simulink model "TwoLevelConverterIdealExample_Pejovic"  (R2023b)
settings: Solver=FixedStepDiscrete  StartTime=0.0  StopTime=100/fsw  MaxStep=1e-4  RelTol=1e-6  AbsTol=1e-6
PreLoadFcn:
  | ts = 1e-5; % local solver sample period
  | fsw = 1e3; % switching frequency
undefined symbols (not defined in the file): DiscIntNeverNeededParam, subcycleFactor
libraries: nesl_utility x53, fl_lib x52, ee_lib x16, simulink x12, fpga_utils_lib x12, eePwmGeneratorTwoLevel x1
(part 1 of 2)
CloseFcn:
  | clear ts fsw;
settings Model: DataTypeOverride=Off  Creator=The MathWorks, Inc.  LastModifiedBy=promero
settings SolverCC: AutoScaleAbsTol=off  AlgebraicLoopSolver=TrustRegion
settings DataIOCC: LimitDataPoints=on  SaveFormat=StructureWithTime  SaveOutput=off  DSMLogging=off  SaveTime=off  ReturnWorkspaceOutputs=off
settings OptimizationCC: BlockReduction=off  ConditionallyExecuteInputs=off  DefaultParameterBehavior=Inlined  OptimizeBlockIOStorage=off  BufferReuse=off  GlobalBufferReuse=off  ExpressionFolding=off  LocalBlockOutputs=off  OptimizeDataStoreBuffers=off  BusAssignmentInplaceUpdate=off
settings DebuggingCC: AlgebraicLoopMsg=error  SolverPrmCheckMsg=warning  SingleTaskRateTransMsg=error  UnconnectedInputMsg=warning  UnconnectedOutputMsg=warning  UnconnectedLineMsg=warning  AllowSymbolicDim=off  PregeneratedLibrarySubsystemCodeDiagnostic=none  SFUnexpectedBacktrackingDiag=warning  SFNoUnconditionalDefaultTransitionDiag=warning  SFExecutionAtInitializationDiag=none  ArithmeticOperatorsInVariantConditions=warning
settings HardwareCC: ProdBitPerPointer=32  ProdBitPerSizeT=32  ProdBitPerPtrDiffT=32  ProdLargestAtomicFloat=None  ProdIntDivRoundTo=Undefined  ProdEndianess=Unspecified  ProdWordSize=32  ProdHWDeviceType=ASIC/FPGA->ASIC/FPGA  TargetBitPerPointer=64  TargetBitPerSizeT=64  TargetBitPerPtrDiffT=64  TargetLongLongMode=on  TargetIntDivRoundTo=Zero  TargetEndianess=LittleEndian  TargetWordSize=64  TargetHWDeviceType=Custom Processor->MATLAB Host Computer  ProdEqTarget=off
settings ModelReferenceCC: EnableRefExpFcnMdlSchedulingChecks=on  PropagateSignalLabelsOutOfModel=off
settings SFSimCC: SimUseLocalCustomCode=off  CustomCodeUndefinedFunction=UseInterfaceOnly
settings RTWCC: RTWUseLocalCustomCode=off  RTWCompilerOptimization=on
settings CodeAppCC: StateflowObjectComments=on
settings GRTTargetCC: TargetLangStandard=C89/C90 (ANSI)
settings ConfigComp: CovMetricSettings=dw  CovSaveCumulativeToWorkspaceVar=on  CovSaveSingleToWorkspaceVar=on  CovExternalEMLEnable=off  CovSFcnEnable=off
settings SimscapeCC: SimscapeNormalizeSystem=off  SimscapeNominalValues="[{\"value\":\"10\",\"unit\":\"V\"},{\"value\":\"1\",\"unit\":\"A\"},{\"value\":\"10\",\"unit\":\"N*m\"},{\"value\":\"10\",\"unit\":\"bar\"},{\"value\":\"100\",\"unit\":\"kJ/kg\"},{\"value\":\"1\",\"unit\":\"kW\"},{\"value\":\"300\",\"unit\":\"K\"},{\"value\":\"100\",\"unit\":\"cm^3/s\"},{\"value\":\"1\",\"unit\":\"kN\"},{\"value\":\"1\",\"unit\":\"g/cm^3\"},{\"value\":\"1\",\"unit\":\"l\"},{\"value\":\"1\",\"unit\":\"cm^2\"},{\"value\":\"60\",\"unit\":\"Hz\"}]"  SimscapeLogType=all

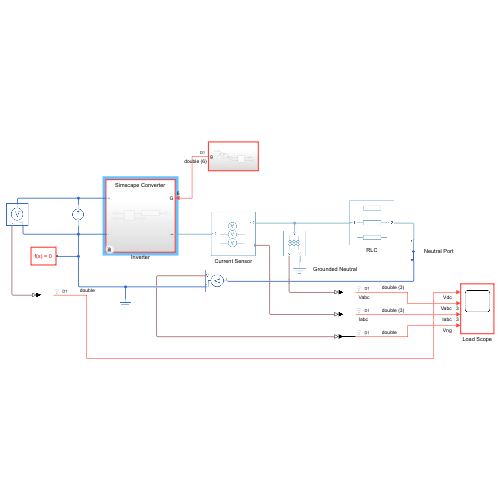
[thumbnail: Simulink's stored preview of the top-level diagram]
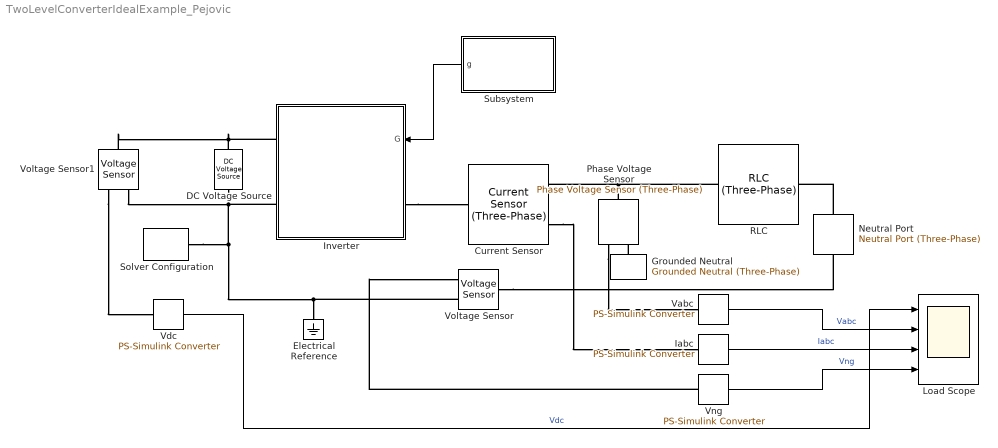
== system TwoLevelConverterIdealExample_Pejovic ==
  Current Sensor : ee_lib/Sensors & Transducers/Current Sensor (Three-Phase)
  DC Voltage Source : fl_lib/Electrical/Electrical Sources/DC Voltage Source  v0=400 V
  Electrical Reference : fl_lib/Electrical/Electrical Elements/Electrical Reference
  Grounded Neutral : ee_lib/Connectors & References/Grounded Neutral (Three-Phase)
  Iabc : nesl_utility/PS-Simulink Converter  PhysicalDomain=network_engine_domain  SubClassName=ps_output  LeftPortType=input  RightPortType=output  PseudoPeriodic=off  Frequencies=[]  VectorFormat=1-D array  Unit=1  AffineConversion=off
  Inverter : Subsystem  Variant=on  VariantControlMode=label  VariantControl=Choice  LabelModeActiveChoice=SimscapeConv
  Load Scope : Scope  NumInputPorts=4
  Neutral Port : ee_lib/Connectors & References/Neutral Port (Three-Phase)  G_parasitic=1e-12 1/Ohm
      settings: InternalSimscapePortConfiguration="{\"Bottom\":[],\"Left\":[{\"id\":\"N\",\"label\":\"~\",\"type\":\"foundation.electrical.three_phase\"}],\"Right\":[{\"id\":\"n\",\"label\":\"n\",\"type\":\"foundation.electrical.electrical\"}],\"Top\":[]}"
  Phase Voltage Sensor : ee_lib/Sensors & Transducers/Phase Voltage Sensor (Three-Phase)
  RLC : ee_lib/Passive/RLC Assemblies/RLC (Three-Phase)  component_structure=4  R=0.1 Ohm  L=0.001 H  C=1e-6 F  R_parasitic=1e-6 Ohm  G_parasitic=1e-6 1/Ohm  IL_specify=on  IL_priority=High  IL=[ 0 0 0 ] A  IL_nominal_specify=off  IL_nominal_unit=A  IL_nominal_value=1  VC_specify=on  VC_priority=High  VC=[ 0 0 0 ] V  VC_nominal_specify=off  VC_nominal_unit=V  VC_nominal_value=1
      settings: InternalSimscapePortConfiguration="{\"Bottom\":[],\"Left\":[{\"id\":\"N1\",\"label\":\"~1\",\"type\":\"foundation.electrical.three_phase\"}],\"Right\":[{\"id\":\"N2\",\"label\":\"~2\",\"type\":\"foundation.electrical.three_phase\"}],\"Top\":[]}"
  Solver Configuration : nesl_utility/Solver Configuration  PhysicalDomain=network_engine_domain  SubClassName=solver  LeftPortType=input  RightPortType=generic  Tones=[]  Harmonics=[]  SimulateNoise=off  Profile=off  UseLocalSampling=off  EnableSwitchedLinearOptims=on  FrequencyDomain=off  UseCCode=off  RelTol=0.001  AbsTol=1e-06  MinStep=1e-09  ToWorkspace=off  RevertToSquareIcSolve=off  NumHomotopyIterations=100  PhasorMode=off  PhasorModeNumHarmonics=1  ConsistencySolver=NEWTON_FTOL  IndexReductionMethod=DerivativeReplacement  DoDC=off  ResidualTolerance=1e-09  ConsistencyTolSource=GLOBAL  ConsistencyAbsTol=0.001  ConsistencyRelTol=0.001  ConsistencyTolFactor=0.001  UseLocalSolver=on  LocalSolverChoice=NE_BACKWARD_EULER_ADVANCER  ResolveIndetEquations=on  FunctionEvalNumThread=1  LocalSolverSampleTime=ts  DoFixedCost=off  MaxNonlinIter=3  MaxModeIter=2  ComputeImpulses=off  ImpulseIterations=2  LinearAlgebra=Sparse  LinearAlgebraNumThread=0  EquationFormulation=NE_TIME_EF  DelaysMemoryBudget=1024  AutomaticFiltering=on  FilteringTimeConstant=0.001  PartitionStorageMethod=AS_NEEDED  PartitionMemoryBudget=1024  PartitionMethod=FAST  MultibodyUseLocalSolver=off  MultibodyLocalSolverChoice=ODE1  MultibodyLocalSolverSampleTime=0.001
  Subsystem : Subsystem
  Vabc : nesl_utility/PS-Simulink Converter  PhysicalDomain=network_engine_domain  SubClassName=ps_output  LeftPortType=input  RightPortType=output  PseudoPeriodic=off  Frequencies=[]  VectorFormat=1-D array  Unit=1  AffineConversion=off
  Vdc : nesl_utility/PS-Simulink Converter  PhysicalDomain=network_engine_domain  SubClassName=ps_output  LeftPortType=input  RightPortType=output  PseudoPeriodic=off  Frequencies=[]  VectorFormat=1-D array  Unit=1  AffineConversion=off
  Vng : nesl_utility/PS-Simulink Converter  PhysicalDomain=network_engine_domain  SubClassName=ps_output  LeftPortType=input  RightPortType=output  PseudoPeriodic=off  Frequencies=[]  VectorFormat=1-D array  Unit=1  AffineConversion=off
  Voltage Sensor : fl_lib/Electrical/Electrical Sensors/Voltage Sensor
  Voltage Sensor1 : fl_lib/Electrical/Electrical Sensors/Voltage Sensor
  wires:
  Vdc/1 -> Load Scope/1  "Vdc"
  Vng/1 -> Load Scope/4  "Vng"
  Vabc/1 -> Load Scope/2  "Vabc"
  Iabc/1 -> Load Scope/3  "Iabc"
  Subsystem/1(g) -> Inverter/1(G)
  connections:
  Voltage Sensor/LConn1 -- Neutral Port/RConn1
  Vng/LConn1 -- Voltage Sensor/RConn1
  Solver Configuration/RConn1 -- Voltage Sensor/RConn2 -- Electrical Reference/LConn1 -- Inverter/RConn2 -- Voltage Sensor1/RConn2 -- DC Voltage Source/RConn1
  Grounded Neutral/LConn1 -- Phase Voltage Sensor/RConn2
  Neutral Port/LConn1 -- RLC/RConn1
  Phase Voltage Sensor/LConn1 -- RLC/LConn1 -- Current Sensor/RConn2
  Current Sensor/RConn1 -- Iabc/LConn1
  Voltage Sensor1/RConn1 -- Vdc/LConn1
  Phase Voltage Sensor/RConn1 -- Vabc/LConn1
  DC Voltage Source/LConn1 -- Inverter/RConn1 -- Voltage Sensor1/LConn1
  Inverter/LConn1 -- Current Sensor/LConn1

== system TwoLevelConverterIdealExample_Pejovic/Inverter ==
  G : Inport
  Pejovic : Subsystem  VariantControl=Pejovic
  Pejovic w/SCA : Subsystem  VariantControl=PejovicSCA
  Simscape Converter : Subsystem  VariantControl=SimscapeConv
  Simscape Switches : Subsystem  VariantControl=SimscapeSw
  + : PMIOPort  Side=Right
  - : PMIOPort  Port=2  Side=Right
  ~ : PMIOPort  Port=3  Side=Left

== system TwoLevelConverterIdealExample_Pejovic/Subsystem ==
  3-ph Unit Sine Wave : Sin  Frequency=2*pi*60  Phase="[0  -2*pi/3  2*pi/3] + pi/2"  SampleTime=ts
  Manual Switch1 : ManualSwitch  CurrentSetting=0
  Mod. Index : Gain  Gain=0.8
  "PWM Generator (Three-phase, Two-level)" : eePwmGeneratorTwoLevel/PWM Generator (Three-phase, Two-level)  PWMMode=Continuous PWM (CPWM)  CPWMMode=SVM: space vector modulation  DPWMMode=120 DPWM: positive dc component  fsw=fsw  Ts=ts
  Product : Product
  SPWM max. input : Constant  Value=400/2
  Terminator : Terminator
  Vdc : Constant  Value=400
  other PWM max. input : Constant  Value=400/sqrt(3)
  g : Outport
  wires:
  "PWM Generator (Three-phase, Two-level)"/1 -> g/1
  Product/1 -> "PWM Generator (Three-phase, Two-level)"/1  "Reference voltages"
  Vdc/1 -> "PWM Generator (Three-phase, Two-level)"/2
  other PWM max. input/1 -> Manual Switch1/2
  SPWM max. input/1 -> Manual Switch1/1
  Manual Switch1/1 -> Mod. Index/1
  "PWM Generator (Three-phase, Two-level)"/2 -> Terminator/1  "Modulation waveforms"
  Mod. Index/1 -> Product/1
  3-ph Unit Sine Wave/1 -> Product/2

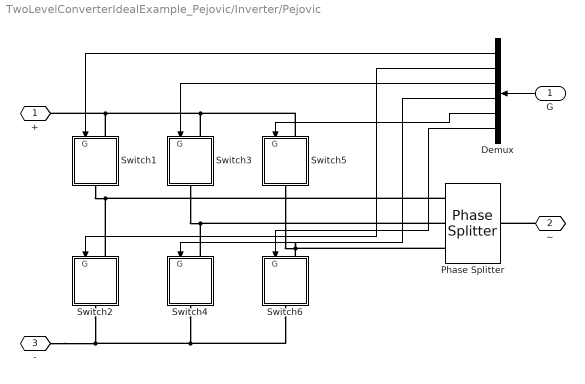
== system TwoLevelConverterIdealExample_Pejovic/Inverter/Pejovic ==
  G : Inport
  Demux : Demux  Outputs=6
  Phase Splitter : ee_lib/Connectors & References/Phase Splitter
  Switch1 : Subsystem  mask{threshold=0.5, Gs=1, timeScaling=1, avgFactor=1}
      mask prompts: threshold "Threshold voltage [V]"; Gs "Conductance (1/Ohm)"; timeScaling "Time scaling"; avgFactor "Subcycle average factor"
      settings: CopyFcn=set_param(gcb, 'LinkStatus', 'none');
  Switch2 : Subsystem  mask{threshold=0.5, Gs=1, timeScaling=1, avgFactor=1}
      mask prompts: threshold "Threshold voltage [V]"; Gs "Conductance (1/Ohm)"; timeScaling "Time scaling"; avgFactor "Subcycle average factor"
      settings: CopyFcn=set_param(gcb, 'LinkStatus', 'none');
  Switch3 : Subsystem  mask{threshold=0.5, Gs=1, timeScaling=1, avgFactor=1}
      mask prompts: threshold "Threshold voltage [V]"; Gs "Conductance (1/Ohm)"; timeScaling "Time scaling"; avgFactor "Subcycle average factor"
      settings: CopyFcn=set_param(gcb, 'LinkStatus', 'none');
  Switch4 : Subsystem  mask{threshold=0.5, Gs=1, timeScaling=1, avgFactor=1}
      mask prompts: threshold "Threshold voltage [V]"; Gs "Conductance (1/Ohm)"; timeScaling "Time scaling"; avgFactor "Subcycle average factor"
      settings: CopyFcn=set_param(gcb, 'LinkStatus', 'none');
  Switch5 : Subsystem  mask{threshold=0.5, Gs=1, timeScaling=1, avgFactor=1}
      mask prompts: threshold "Threshold voltage [V]"; Gs "Conductance (1/Ohm)"; timeScaling "Time scaling"; avgFactor "Subcycle average factor"
      settings: CopyFcn=set_param(gcb, 'LinkStatus', 'none');
  Switch6 : Subsystem  mask{threshold=0.5, Gs=1, timeScaling=1, avgFactor=1}
      mask prompts: threshold "Threshold voltage [V]"; Gs "Conductance (1/Ohm)"; timeScaling "Time scaling"; avgFactor "Subcycle average factor"
      settings: CopyFcn=set_param(gcb, 'LinkStatus', 'none');
  + : PMIOPort  Side=Right
  ~ : PMIOPort  Port=2  Side=Left
  - : PMIOPort  Port=3  Side=Right
  wires:
  Demux/6 -> Switch6/1(G)
  Demux/5 -> Switch5/1(G)
  Demux/4 -> Switch4/1(G)
  Demux/3 -> Switch3/1(G)
  Demux/2 -> Switch2/1(G)
  Demux/1 -> Switch1/1(G)
  G/1 -> Demux/1
  connections:
  +/RConn1 -- Switch1/LConn1 -- Switch5/LConn1 -- Switch3/LConn1
  Phase Splitter/RConn1 -- Switch2/LConn1 -- Switch1/RConn1
  Switch6/RConn1 -- Switch4/RConn1 -- Switch2/RConn1 -- -/RConn1
  ~/RConn1 -- Phase Splitter/LConn1
  Phase Splitter/RConn2 -- Switch4/LConn1 -- Switch3/RConn1
  Phase Splitter/RConn3 -- Switch6/LConn1 -- Switch5/RConn1

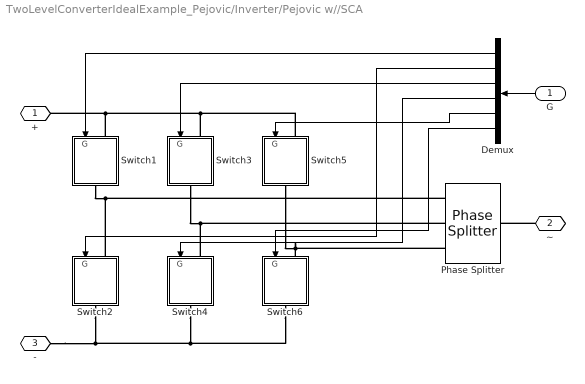
== system TwoLevelConverterIdealExample_Pejovic/Inverter/Pejovic w//SCA ==
  G : Inport
  Demux : Demux  Outputs=6
  Phase Splitter : ee_lib/Connectors & References/Phase Splitter
  Switch1 : Subsystem  mask{threshold=0.5, Gs=1, timeScaling=1, avgFactor=subcycleFactor}
      mask prompts: threshold "Threshold voltage [V]"; Gs "Conductance (1/Ohm)"; timeScaling "Time scaling"; avgFactor "Subcycle average factor"
      settings: CopyFcn=set_param(gcb, 'LinkStatus', 'none');
  Switch2 : Subsystem  mask{threshold=0.5, Gs=1, timeScaling=1, avgFactor=subcycleFactor}
      mask prompts: threshold "Threshold voltage [V]"; Gs "Conductance (1/Ohm)"; timeScaling "Time scaling"; avgFactor "Subcycle average factor"
      settings: CopyFcn=set_param(gcb, 'LinkStatus', 'none');
  Switch3 : Subsystem  mask{threshold=0.5, Gs=1, timeScaling=1, avgFactor=subcycleFactor}
      mask prompts: threshold "Threshold voltage [V]"; Gs "Conductance (1/Ohm)"; timeScaling "Time scaling"; avgFactor "Subcycle average factor"
      settings: CopyFcn=set_param(gcb, 'LinkStatus', 'none');
  Switch4 : Subsystem  mask{threshold=0.5, Gs=1, timeScaling=1, avgFactor=subcycleFactor}
      mask prompts: threshold "Threshold voltage [V]"; Gs "Conductance (1/Ohm)"; timeScaling "Time scaling"; avgFactor "Subcycle average factor"
      settings: CopyFcn=set_param(gcb, 'LinkStatus', 'none');
  Switch5 : Subsystem  mask{threshold=0.5, Gs=1, timeScaling=1, avgFactor=subcycleFactor}
      mask prompts: threshold "Threshold voltage [V]"; Gs "Conductance (1/Ohm)"; timeScaling "Time scaling"; avgFactor "Subcycle average factor"
      settings: CopyFcn=set_param(gcb, 'LinkStatus', 'none');
  Switch6 : Subsystem  mask{threshold=0.5, Gs=1, timeScaling=1, avgFactor=subcycleFactor}
      mask prompts: threshold "Threshold voltage [V]"; Gs "Conductance (1/Ohm)"; timeScaling "Time scaling"; avgFactor "Subcycle average factor"
      settings: CopyFcn=set_param(gcb, 'LinkStatus', 'none');
  + : PMIOPort  Side=Right
  ~ : PMIOPort  Port=2  Side=Left
  - : PMIOPort  Port=3  Side=Right
  wires:
  G/1 -> Demux/1
  Demux/1 -> Switch1/1(G)
  Demux/2 -> Switch2/1(G)
  Demux/3 -> Switch3/1(G)
  Demux/4 -> Switch4/1(G)
  Demux/5 -> Switch5/1(G)
  Demux/6 -> Switch6/1(G)
  connections:
  Switch6/LConn1 -- Phase Splitter/RConn3 -- Switch5/RConn1
  Switch4/LConn1 -- Phase Splitter/RConn2 -- Switch3/RConn1
  ~/RConn1 -- Phase Splitter/LConn1
  Switch6/RConn1 -- -/RConn1 -- Switch2/RConn1 -- Switch4/RConn1
  Switch2/LConn1 -- Phase Splitter/RConn1 -- Switch1/RConn1
  Switch5/LConn1 -- +/RConn1 -- Switch1/LConn1 -- Switch3/LConn1

== system TwoLevelConverterIdealExample_Pejovic/Inverter/Simscape Converter ==
  G : Inport
  Converter (Three-Phase) : ee_lib/Semiconductors & Converters/Converters/Converter (Three-Phase)  port_option=ee.enum.threePhasePort.composite  device_type=ee.enum.converters.switchingdevice.ideal  K=0  Vf=0.8 V  Ron=0.001 Ohm  Rds=0.001 Ohm  Goff=1e-6 1/Ohm  Vgt=1 V  Vgt_off=-1 V  Ih=1 A  Vth=0.5 V  diode_param=ee.enum.converters.protectiondiode.none  diode_Vf=0.8 V  diode_Ron=0.001 Ohm  diode_Goff=1e-5 1/Ohm  diode_C=50 nF  diode_iRM=-235 A  diode_iF=300 A  diode_idot=-50 A/us  diode_trr_param=ee.enum.converters.diodetrr.trr_factor  diode_trr_factor=3  diode_trr=15 us  diode_Qrr=1500 s*uA  snubber_type=ee.enum.converters.snubber.exclude  Cs=1e-7 F  Rs=0.1 Ohm
  Gates : Subsystem
  + : PMIOPort  Side=Right
  ~ : PMIOPort  Port=2  Side=Left
  - : PMIOPort  Port=3  Side=Right
  wires:
  G/1 -> Gates/1(Gates Simulink)
  connections:
  -/RConn1 -- Converter (Three-Phase)/RConn2
  Converter (Three-Phase)/RConn1 -- +/RConn1
  Gates/RConn1 -- Converter (Three-Phase)/LConn1
  Converter (Three-Phase)/LConn2 -- ~/RConn1

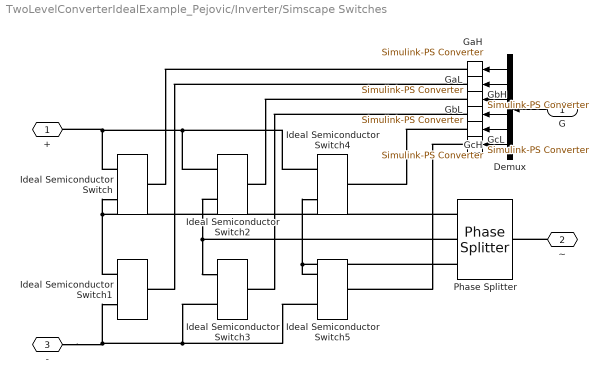
== system TwoLevelConverterIdealExample_Pejovic/Inverter/Simscape Switches ==
  G : Inport
  Demux : Demux  Outputs=6
  GaH : nesl_utility/Simulink-PS Converter  PhysicalDomain=network_engine_domain  SubClassName=ps_input  LeftPortType=input  RightPortType=output  PseudoPeriodic=off  Frequencies=[]  NoiseDistribution=none  NoiseParameters=[]  Unit=1  AffineConversion=off  FilteringAndDerivatives=zero  SimscapeFilterOrder=1  InputFilterTimeConstant=0.001  UdotUserProvided=0
  GaL : nesl_utility/Simulink-PS Converter  PhysicalDomain=network_engine_domain  SubClassName=ps_input  LeftPortType=input  RightPortType=output  PseudoPeriodic=off  Frequencies=[]  NoiseDistribution=none  NoiseParameters=[]  Unit=1  AffineConversion=off  FilteringAndDerivatives=zero  SimscapeFilterOrder=1  InputFilterTimeConstant=0.001  UdotUserProvided=0
  GbH : nesl_utility/Simulink-PS Converter  PhysicalDomain=network_engine_domain  SubClassName=ps_input  LeftPortType=input  RightPortType=output  PseudoPeriodic=off  Frequencies=[]  NoiseDistribution=none  NoiseParameters=[]  Unit=1  AffineConversion=off  FilteringAndDerivatives=zero  SimscapeFilterOrder=1  InputFilterTimeConstant=0.001  UdotUserProvided=0
  GbL : nesl_utility/Simulink-PS Converter  PhysicalDomain=network_engine_domain  SubClassName=ps_input  LeftPortType=input  RightPortType=output  PseudoPeriodic=off  Frequencies=[]  NoiseDistribution=none  NoiseParameters=[]  Unit=1  AffineConversion=off  FilteringAndDerivatives=zero  SimscapeFilterOrder=1  InputFilterTimeConstant=0.001  UdotUserProvided=0
  GcH : nesl_utility/Simulink-PS Converter  PhysicalDomain=network_engine_domain  SubClassName=ps_input  LeftPortType=input  RightPortType=output  PseudoPeriodic=off  Frequencies=[]  NoiseDistribution=none  NoiseParameters=[]  Unit=1  AffineConversion=off  FilteringAndDerivatives=zero  SimscapeFilterOrder=1  InputFilterTimeConstant=0.001  UdotUserProvided=0
  GcL : nesl_utility/Simulink-PS Converter  PhysicalDomain=network_engine_domain  SubClassName=ps_input  LeftPortType=input  RightPortType=output  PseudoPeriodic=off  Frequencies=[]  NoiseDistribution=none  NoiseParameters=[]  Unit=1  AffineConversion=off  FilteringAndDerivatives=zero  SimscapeFilterOrder=1  InputFilterTimeConstant=0.001  UdotUserProvided=0
  Ideal Semiconductor Switch{,1..5} (6 alike) : ee_lib/Semiconductors & Converters/Ideal Semiconductor Switch  port_option=ee.enum.controlport.ps  Ron=0.001 Ohm  Goff=1e-6 1/Ohm  Vth=0.5 V  diode_param=ee.enum.converters.protectiondiode.none  diode_Vf=0.8 V  diode_Ron=0.001 Ohm  diode_Goff=1e-5 1/Ohm  diode_C=50e-9 F  diode_iRM=-235 A  diode_iF=300 A  diode_idot=-50 A/us  diode_trr_param=ee.enum.converters.diodetrr.trr_factor  diode_trr_factor=3  diode_trr=15 us  diode_Qrr=1500 s*uA
  Phase Splitter : ee_lib/Connectors & References/Phase Splitter
  + : PMIOPort  Side=Right
  ~ : PMIOPort  Port=2  Side=Left
  - : PMIOPort  Port=3  Side=Right
  wires:
  Demux/6 -> GcL/1
  Demux/2 -> GaL/1
  Demux/3 -> GbH/1
  Demux/5 -> GcH/1
  Demux/4 -> GbL/1
  Demux/1 -> GaH/1
  G/1 -> Demux/1
  connections:
  Ideal Semiconductor Switch/RConn1 -- Ideal Semiconductor Switch4/RConn1 -- Ideal Semiconductor Switch2/RConn1 -- +/RConn1
  Ideal Semiconductor Switch1/RConn1 -- Phase Splitter/RConn1 -- Ideal Semiconductor Switch/RConn2
  -/RConn1 -- Ideal Semiconductor Switch5/RConn2 -- Ideal Semiconductor Switch3/RConn2 -- Ideal Semiconductor Switch1/RConn2
  ~/RConn1 -- Phase Splitter/LConn1
  Ideal Semiconductor Switch2/RConn2 -- Ideal Semiconductor Switch3/RConn1 -- Phase Splitter/RConn2
  Ideal Semiconductor Switch5/RConn1 -- Ideal Semiconductor Switch4/RConn2 -- Phase Splitter/RConn3
  GaH/RConn1 -- Ideal Semiconductor Switch/LConn1
  GaL/RConn1 -- Ideal Semiconductor Switch1/LConn1
  GbH/RConn1 -- Ideal Semiconductor Switch2/LConn1
  GbL/RConn1 -- Ideal Semiconductor Switch3/LConn1
  GcH/RConn1 -- Ideal Semiconductor Switch4/LConn1
  GcL/RConn1 -- Ideal Semiconductor Switch5/LConn1

== system TwoLevelConverterIdealExample_Pejovic/Inverter/Pejovic/Switch1 ==
  G : Inport
  Controller : Subsystem  mask{threshold=threshold, Gs=Gs, s=timeScaling, avgFactor=avgFactor}
      mask prompts: Gs "Conductance (1/Ohm)"; s "Time scaling"; avgFactor "Subcycle average factor"
      mask DialogControl DescGroupVar Prompt: Description
      mask DialogControl Details Prompt: Switch Controller
  Gs : fl_lib/Electrical/Electrical Elements/Resistor  R=1/Gs Ohm  i_specify=off  i_priority=None  i=0 A  i_nominal_specify=off  i_nominal_unit=A  i_nominal_value=1  v_specify=off  v_priority=None  v=0 V  v_nominal_specify=off  v_nominal_unit=V  v_nominal_value=1
      settings: LibrarySourceBlock=SimscapeFPGAHIL_lib/Linearized Switch Models/Switch/Gs
  ic : fl_lib/Electrical/Electrical Sources/Controlled Current Source
      settings: LibrarySourceBlock=SimscapeFPGAHIL_lib/Linearized Switch Models/Switch/ic
  ic_in : nesl_utility/Simulink-PS Converter  PhysicalDomain=network_engine_domain  SubClassName=ps_input  LeftPortType=input  RightPortType=output  PseudoPeriodic=off  Frequencies=[]  NoiseDistribution=none  NoiseParameters=[]  Unit=A  AffineConversion=off  FilteringAndDerivatives=provide  SimscapeFilterOrder=1  InputFilterTimeConstant=0.001  UdotUserProvided=0
      settings: LibrarySourceBlock=SimscapeFPGAHIL_lib/Linearized Switch Models/Switch/ic_in
  is : fl_lib/Electrical/Electrical Sensors/Current Sensor
      settings: LibrarySourceBlock=SimscapeFPGAHIL_lib/Linearized Switch Models/Switch/is
  is_out : nesl_utility/PS-Simulink Converter  PhysicalDomain=network_engine_domain  SubClassName=ps_output  LeftPortType=input  RightPortType=output  PseudoPeriodic=off  Frequencies=[]  VectorFormat=1-D array  Unit=A  AffineConversion=off
      settings: LibrarySourceBlock=SimscapeFPGAHIL_lib/Linearized Switch Models/Switch/is_out
  vs : fl_lib/Electrical/Electrical Sensors/Voltage Sensor
      settings: LibrarySourceBlock=SimscapeFPGAHIL_lib/Linearized Switch Models/Switch/vs
  vs_out : nesl_utility/PS-Simulink Converter  PhysicalDomain=network_engine_domain  SubClassName=ps_output  LeftPortType=input  RightPortType=output  PseudoPeriodic=off  Frequencies=[]  VectorFormat=1-D array  Unit=V  AffineConversion=off
      settings: LibrarySourceBlock=SimscapeFPGAHIL_lib/Linearized Switch Models/Switch/vs_out
  + : PMIOPort  Side=Left
  - : PMIOPort  Port=2  Side=Right
  wires:
  vs_out/1 -> Controller/1(vs)
  is_out/1 -> Controller/2(is)
  G/1 -> Controller/3(G)
  Controller/1(ic) -> ic_in/1
  connections:
  ic/LConn1 -- Gs/LConn1 -- is/RConn2
  vs/RConn2 -- -/RConn1 -- Gs/RConn1 -- ic/RConn2
  vs/LConn1 -- +/RConn1 -- is/LConn1
  ic_in/RConn1 -- ic/RConn1
  vs_out/LConn1 -- vs/RConn1
  is_out/LConn1 -- is/RConn1

== system TwoLevelConverterIdealExample_Pejovic/Inverter/Pejovic/Switch2 ==
  G : Inport
  Controller : Subsystem  mask{threshold=threshold, Gs=Gs, s=timeScaling, avgFactor=avgFactor}
      mask prompts: Gs "Conductance (1/Ohm)"; s "Time scaling"; avgFactor "Subcycle average factor"
      mask DialogControl DescGroupVar Prompt: Description
      mask DialogControl Details Prompt: Switch Controller
  Gs : fl_lib/Electrical/Electrical Elements/Resistor  R=1/Gs Ohm  i_specify=off  i_priority=None  i=0 A  i_nominal_specify=off  i_nominal_unit=A  i_nominal_value=1  v_specify=off  v_priority=None  v=0 V  v_nominal_specify=off  v_nominal_unit=V  v_nominal_value=1
      settings: LibrarySourceBlock=SimscapeFPGAHIL_lib/Linearized Switch Models/Switch/Gs
  ic : fl_lib/Electrical/Electrical Sources/Controlled Current Source
      settings: LibrarySourceBlock=SimscapeFPGAHIL_lib/Linearized Switch Models/Switch/ic
  ic_in : nesl_utility/Simulink-PS Converter  PhysicalDomain=network_engine_domain  SubClassName=ps_input  LeftPortType=input  RightPortType=output  PseudoPeriodic=off  Frequencies=[]  NoiseDistribution=none  NoiseParameters=[]  Unit=A  AffineConversion=off  FilteringAndDerivatives=provide  SimscapeFilterOrder=1  InputFilterTimeConstant=0.001  UdotUserProvided=0
      settings: LibrarySourceBlock=SimscapeFPGAHIL_lib/Linearized Switch Models/Switch/ic_in
  is : fl_lib/Electrical/Electrical Sensors/Current Sensor
      settings: LibrarySourceBlock=SimscapeFPGAHIL_lib/Linearized Switch Models/Switch/is
  is_out : nesl_utility/PS-Simulink Converter  PhysicalDomain=network_engine_domain  SubClassName=ps_output  LeftPortType=input  RightPortType=output  PseudoPeriodic=off  Frequencies=[]  VectorFormat=1-D array  Unit=A  AffineConversion=off
      settings: LibrarySourceBlock=SimscapeFPGAHIL_lib/Linearized Switch Models/Switch/is_out
  vs : fl_lib/Electrical/Electrical Sensors/Voltage Sensor
      settings: LibrarySourceBlock=SimscapeFPGAHIL_lib/Linearized Switch Models/Switch/vs
  vs_out : nesl_utility/PS-Simulink Converter  PhysicalDomain=network_engine_domain  SubClassName=ps_output  LeftPortType=input  RightPortType=output  PseudoPeriodic=off  Frequencies=[]  VectorFormat=1-D array  Unit=V  AffineConversion=off
      settings: LibrarySourceBlock=SimscapeFPGAHIL_lib/Linearized Switch Models/Switch/vs_out
  + : PMIOPort  Side=Left
  - : PMIOPort  Port=2  Side=Right
  wires:
  Controller/1(ic) -> ic_in/1
  G/1 -> Controller/3(G)
  is_out/1 -> Controller/2(is)
  vs_out/1 -> Controller/1(vs)
  connections:
  is_out/LConn1 -- is/RConn1
  vs_out/LConn1 -- vs/RConn1
  ic_in/RConn1 -- ic/RConn1
  is/LConn1 -- +/RConn1 -- vs/LConn1
  ic/RConn2 -- Gs/RConn1 -- -/RConn1 -- vs/RConn2
  is/RConn2 -- Gs/LConn1 -- ic/LConn1

== system TwoLevelConverterIdealExample_Pejovic/Inverter/Pejovic/Switch3 ==
  G : Inport
  Controller : Subsystem  mask{threshold=threshold, Gs=Gs, s=timeScaling, avgFactor=avgFactor}
      mask prompts: Gs "Conductance (1/Ohm)"; s "Time scaling"; avgFactor "Subcycle average factor"
      mask DialogControl DescGroupVar Prompt: Description
      mask DialogControl Details Prompt: Switch Controller
  Gs : fl_lib/Electrical/Electrical Elements/Resistor  R=1/Gs Ohm  i_specify=off  i_priority=None  i=0 A  i_nominal_specify=off  i_nominal_unit=A  i_nominal_value=1  v_specify=off  v_priority=None  v=0 V  v_nominal_specify=off  v_nominal_unit=V  v_nominal_value=1
      settings: LibrarySourceBlock=SimscapeFPGAHIL_lib/Linearized Switch Models/Switch/Gs
  ic : fl_lib/Electrical/Electrical Sources/Controlled Current Source
      settings: LibrarySourceBlock=SimscapeFPGAHIL_lib/Linearized Switch Models/Switch/ic
  ic_in : nesl_utility/Simulink-PS Converter  PhysicalDomain=network_engine_domain  SubClassName=ps_input  LeftPortType=input  RightPortType=output  PseudoPeriodic=off  Frequencies=[]  NoiseDistribution=none  NoiseParameters=[]  Unit=A  AffineConversion=off  FilteringAndDerivatives=provide  SimscapeFilterOrder=1  InputFilterTimeConstant=0.001  UdotUserProvided=0
      settings: LibrarySourceBlock=SimscapeFPGAHIL_lib/Linearized Switch Models/Switch/ic_in
  is : fl_lib/Electrical/Electrical Sensors/Current Sensor
      settings: LibrarySourceBlock=SimscapeFPGAHIL_lib/Linearized Switch Models/Switch/is
  is_out : nesl_utility/PS-Simulink Converter  PhysicalDomain=network_engine_domain  SubClassName=ps_output  LeftPortType=input  RightPortType=output  PseudoPeriodic=off  Frequencies=[]  VectorFormat=1-D array  Unit=A  AffineConversion=off
      settings: LibrarySourceBlock=SimscapeFPGAHIL_lib/Linearized Switch Models/Switch/is_out
  vs : fl_lib/Electrical/Electrical Sensors/Voltage Sensor
      settings: LibrarySourceBlock=SimscapeFPGAHIL_lib/Linearized Switch Models/Switch/vs
  vs_out : nesl_utility/PS-Simulink Converter  PhysicalDomain=network_engine_domain  SubClassName=ps_output  LeftPortType=input  RightPortType=output  PseudoPeriodic=off  Frequencies=[]  VectorFormat=1-D array  Unit=V  AffineConversion=off
      settings: LibrarySourceBlock=SimscapeFPGAHIL_lib/Linearized Switch Models/Switch/vs_out
  + : PMIOPort  Side=Left
  - : PMIOPort  Port=2  Side=Right
  wires:
  vs_out/1 -> Controller/1(vs)
  is_out/1 -> Controller/2(is)
  G/1 -> Controller/3(G)
  Controller/1(ic) -> ic_in/1
  connections:
  ic/LConn1 -- Gs/LConn1 -- is/RConn2
  vs/RConn2 -- -/RConn1 -- Gs/RConn1 -- ic/RConn2
  vs/LConn1 -- +/RConn1 -- is/LConn1
  ic_in/RConn1 -- ic/RConn1
  vs_out/LConn1 -- vs/RConn1
  is_out/LConn1 -- is/RConn1

== system TwoLevelConverterIdealExample_Pejovic/Inverter/Pejovic/Switch4 ==
  G : Inport
  Controller : Subsystem  mask{threshold=threshold, Gs=Gs, s=timeScaling, avgFactor=avgFactor}
      mask prompts: Gs "Conductance (1/Ohm)"; s "Time scaling"; avgFactor "Subcycle average factor"
      mask DialogControl DescGroupVar Prompt: Description
      mask DialogControl Details Prompt: Switch Controller
  Gs : fl_lib/Electrical/Electrical Elements/Resistor  R=1/Gs Ohm  i_specify=off  i_priority=None  i=0 A  i_nominal_specify=off  i_nominal_unit=A  i_nominal_value=1  v_specify=off  v_priority=None  v=0 V  v_nominal_specify=off  v_nominal_unit=V  v_nominal_value=1
      settings: LibrarySourceBlock=SimscapeFPGAHIL_lib/Linearized Switch Models/Switch/Gs
  ic : fl_lib/Electrical/Electrical Sources/Controlled Current Source
      settings: LibrarySourceBlock=SimscapeFPGAHIL_lib/Linearized Switch Models/Switch/ic
  ic_in : nesl_utility/Simulink-PS Converter  PhysicalDomain=network_engine_domain  SubClassName=ps_input  LeftPortType=input  RightPortType=output  PseudoPeriodic=off  Frequencies=[]  NoiseDistribution=none  NoiseParameters=[]  Unit=A  AffineConversion=off  FilteringAndDerivatives=provide  SimscapeFilterOrder=1  InputFilterTimeConstant=0.001  UdotUserProvided=0
      settings: LibrarySourceBlock=SimscapeFPGAHIL_lib/Linearized Switch Models/Switch/ic_in
  is : fl_lib/Electrical/Electrical Sensors/Current Sensor
      settings: LibrarySourceBlock=SimscapeFPGAHIL_lib/Linearized Switch Models/Switch/is
  is_out : nesl_utility/PS-Simulink Converter  PhysicalDomain=network_engine_domain  SubClassName=ps_output  LeftPortType=input  RightPortType=output  PseudoPeriodic=off  Frequencies=[]  VectorFormat=1-D array  Unit=A  AffineConversion=off
      settings: LibrarySourceBlock=SimscapeFPGAHIL_lib/Linearized Switch Models/Switch/is_out
  vs : fl_lib/Electrical/Electrical Sensors/Voltage Sensor
      settings: LibrarySourceBlock=SimscapeFPGAHIL_lib/Linearized Switch Models/Switch/vs
  vs_out : nesl_utility/PS-Simulink Converter  PhysicalDomain=network_engine_domain  SubClassName=ps_output  LeftPortType=input  RightPortType=output  PseudoPeriodic=off  Frequencies=[]  VectorFormat=1-D array  Unit=V  AffineConversion=off
      settings: LibrarySourceBlock=SimscapeFPGAHIL_lib/Linearized Switch Models/Switch/vs_out
  + : PMIOPort  Side=Left
  - : PMIOPort  Port=2  Side=Right
  wires:
  Controller/1(ic) -> ic_in/1
  G/1 -> Controller/3(G)
  is_out/1 -> Controller/2(is)
  vs_out/1 -> Controller/1(vs)
  connections:
  is_out/LConn1 -- is/RConn1
  vs_out/LConn1 -- vs/RConn1
  ic_in/RConn1 -- ic/RConn1
  is/LConn1 -- +/RConn1 -- vs/LConn1
  ic/RConn2 -- Gs/RConn1 -- -/RConn1 -- vs/RConn2
  is/RConn2 -- Gs/LConn1 -- ic/LConn1

== system TwoLevelConverterIdealExample_Pejovic/Inverter/Pejovic/Switch5 ==
  G : Inport
  Controller : Subsystem  mask{threshold=threshold, Gs=Gs, s=timeScaling, avgFactor=avgFactor}
      mask prompts: Gs "Conductance (1/Ohm)"; s "Time scaling"; avgFactor "Subcycle average factor"
      mask DialogControl DescGroupVar Prompt: Description
      mask DialogControl Details Prompt: Switch Controller
  Gs : fl_lib/Electrical/Electrical Elements/Resistor  R=1/Gs Ohm  i_specify=off  i_priority=None  i=0 A  i_nominal_specify=off  i_nominal_unit=A  i_nominal_value=1  v_specify=off  v_priority=None  v=0 V  v_nominal_specify=off  v_nominal_unit=V  v_nominal_value=1
      settings: LibrarySourceBlock=SimscapeFPGAHIL_lib/Linearized Switch Models/Switch/Gs
  ic : fl_lib/Electrical/Electrical Sources/Controlled Current Source
      settings: LibrarySourceBlock=SimscapeFPGAHIL_lib/Linearized Switch Models/Switch/ic
  ic_in : nesl_utility/Simulink-PS Converter  PhysicalDomain=network_engine_domain  SubClassName=ps_input  LeftPortType=input  RightPortType=output  PseudoPeriodic=off  Frequencies=[]  NoiseDistribution=none  NoiseParameters=[]  Unit=A  AffineConversion=off  FilteringAndDerivatives=provide  SimscapeFilterOrder=1  InputFilterTimeConstant=0.001  UdotUserProvided=0
      settings: LibrarySourceBlock=SimscapeFPGAHIL_lib/Linearized Switch Models/Switch/ic_in
  is : fl_lib/Electrical/Electrical Sensors/Current Sensor
      settings: LibrarySourceBlock=SimscapeFPGAHIL_lib/Linearized Switch Models/Switch/is
  is_out : nesl_utility/PS-Simulink Converter  PhysicalDomain=network_engine_domain  SubClassName=ps_output  LeftPortType=input  RightPortType=output  PseudoPeriodic=off  Frequencies=[]  VectorFormat=1-D array  Unit=A  AffineConversion=off
      settings: LibrarySourceBlock=SimscapeFPGAHIL_lib/Linearized Switch Models/Switch/is_out
  vs : fl_lib/Electrical/Electrical Sensors/Voltage Sensor
      settings: LibrarySourceBlock=SimscapeFPGAHIL_lib/Linearized Switch Models/Switch/vs
  vs_out : nesl_utility/PS-Simulink Converter  PhysicalDomain=network_engine_domain  SubClassName=ps_output  LeftPortType=input  RightPortType=output  PseudoPeriodic=off  Frequencies=[]  VectorFormat=1-D array  Unit=V  AffineConversion=off
      settings: LibrarySourceBlock=SimscapeFPGAHIL_lib/Linearized Switch Models/Switch/vs_out
  + : PMIOPort  Side=Left
  - : PMIOPort  Port=2  Side=Right
  wires:
  vs_out/1 -> Controller/1(vs)
  is_out/1 -> Controller/2(is)
  G/1 -> Controller/3(G)
  Controller/1(ic) -> ic_in/1
  connections:
  ic/LConn1 -- Gs/LConn1 -- is/RConn2
  vs/RConn2 -- -/RConn1 -- Gs/RConn1 -- ic/RConn2
  vs/LConn1 -- +/RConn1 -- is/LConn1
  ic_in/RConn1 -- ic/RConn1
  vs_out/LConn1 -- vs/RConn1
  is_out/LConn1 -- is/RConn1

== system TwoLevelConverterIdealExample_Pejovic/Inverter/Pejovic/Switch6 ==
  G : Inport
  Controller : Subsystem  mask{threshold=threshold, Gs=Gs, s=timeScaling, avgFactor=avgFactor}
      mask prompts: Gs "Conductance (1/Ohm)"; s "Time scaling"; avgFactor "Subcycle average factor"
      mask DialogControl DescGroupVar Prompt: Description
      mask DialogControl Details Prompt: Switch Controller
  Gs : fl_lib/Electrical/Electrical Elements/Resistor  R=1/Gs Ohm  i_specify=off  i_priority=None  i=0 A  i_nominal_specify=off  i_nominal_unit=A  i_nominal_value=1  v_specify=off  v_priority=None  v=0 V  v_nominal_specify=off  v_nominal_unit=V  v_nominal_value=1
      settings: LibrarySourceBlock=SimscapeFPGAHIL_lib/Linearized Switch Models/Switch/Gs
  ic : fl_lib/Electrical/Electrical Sources/Controlled Current Source
      settings: LibrarySourceBlock=SimscapeFPGAHIL_lib/Linearized Switch Models/Switch/ic
  ic_in : nesl_utility/Simulink-PS Converter  PhysicalDomain=network_engine_domain  SubClassName=ps_input  LeftPortType=input  RightPortType=output  PseudoPeriodic=off  Frequencies=[]  NoiseDistribution=none  NoiseParameters=[]  Unit=A  AffineConversion=off  FilteringAndDerivatives=provide  SimscapeFilterOrder=1  InputFilterTimeConstant=0.001  UdotUserProvided=0
      settings: LibrarySourceBlock=SimscapeFPGAHIL_lib/Linearized Switch Models/Switch/ic_in
  is : fl_lib/Electrical/Electrical Sensors/Current Sensor
      settings: LibrarySourceBlock=SimscapeFPGAHIL_lib/Linearized Switch Models/Switch/is
  is_out : nesl_utility/PS-Simulink Converter  PhysicalDomain=network_engine_domain  SubClassName=ps_output  LeftPortType=input  RightPortType=output  PseudoPeriodic=off  Frequencies=[]  VectorFormat=1-D array  Unit=A  AffineConversion=off
      settings: LibrarySourceBlock=SimscapeFPGAHIL_lib/Linearized Switch Models/Switch/is_out
  vs : fl_lib/Electrical/Electrical Sensors/Voltage Sensor
      settings: LibrarySourceBlock=SimscapeFPGAHIL_lib/Linearized Switch Models/Switch/vs
  vs_out : nesl_utility/PS-Simulink Converter  PhysicalDomain=network_engine_domain  SubClassName=ps_output  LeftPortType=input  RightPortType=output  PseudoPeriodic=off  Frequencies=[]  VectorFormat=1-D array  Unit=V  AffineConversion=off
      settings: LibrarySourceBlock=SimscapeFPGAHIL_lib/Linearized Switch Models/Switch/vs_out
  + : PMIOPort  Side=Left
  - : PMIOPort  Port=2  Side=Right
  wires:
  Controller/1(ic) -> ic_in/1
  G/1 -> Controller/3(G)
  is_out/1 -> Controller/2(is)
  vs_out/1 -> Controller/1(vs)
  connections:
  is_out/LConn1 -- is/RConn1
  vs_out/LConn1 -- vs/RConn1
  ic_in/RConn1 -- ic/RConn1
  is/LConn1 -- +/RConn1 -- vs/LConn1
  ic/RConn2 -- Gs/RConn1 -- -/RConn1 -- vs/RConn2
  is/RConn2 -- Gs/LConn1 -- ic/LConn1

== system TwoLevelConverterIdealExample_Pejovic/Inverter/Pejovic w//SCA/Switch1 ==
  G : Inport
  Controller : Subsystem  mask{threshold=threshold, Gs=Gs, s=timeScaling, avgFactor=avgFactor}
      mask prompts: Gs "Conductance (1/Ohm)"; s "Time scaling"; avgFactor "Subcycle average factor"
      mask DialogControl DescGroupVar Prompt: Description
      mask DialogControl Details Prompt: Switch Controller
  Gs : fl_lib/Electrical/Electrical Elements/Resistor  R=1/Gs Ohm  i_specify=off  i_priority=None  i=0 A  i_nominal_specify=off  i_nominal_unit=A  i_nominal_value=1  v_specify=off  v_priority=None  v=0 V  v_nominal_specify=off  v_nominal_unit=V  v_nominal_value=1
      settings: LibrarySourceBlock=SimscapeFPGAHIL_lib/Linearized Switch Models/Switch/Gs
  ic : fl_lib/Electrical/Electrical Sources/Controlled Current Source
      settings: LibrarySourceBlock=SimscapeFPGAHIL_lib/Linearized Switch Models/Switch/ic
  ic_in : nesl_utility/Simulink-PS Converter  PhysicalDomain=network_engine_domain  SubClassName=ps_input  LeftPortType=input  RightPortType=output  PseudoPeriodic=off  Frequencies=[]  NoiseDistribution=none  NoiseParameters=[]  Unit=A  AffineConversion=off  FilteringAndDerivatives=provide  SimscapeFilterOrder=1  InputFilterTimeConstant=0.001  UdotUserProvided=0
      settings: LibrarySourceBlock=SimscapeFPGAHIL_lib/Linearized Switch Models/Switch/ic_in
  is : fl_lib/Electrical/Electrical Sensors/Current Sensor
      settings: LibrarySourceBlock=SimscapeFPGAHIL_lib/Linearized Switch Models/Switch/is
  is_out : nesl_utility/PS-Simulink Converter  PhysicalDomain=network_engine_domain  SubClassName=ps_output  LeftPortType=input  RightPortType=output  PseudoPeriodic=off  Frequencies=[]  VectorFormat=1-D array  Unit=A  AffineConversion=off
      settings: LibrarySourceBlock=SimscapeFPGAHIL_lib/Linearized Switch Models/Switch/is_out
  vs : fl_lib/Electrical/Electrical Sensors/Voltage Sensor
      settings: LibrarySourceBlock=SimscapeFPGAHIL_lib/Linearized Switch Models/Switch/vs
  vs_out : nesl_utility/PS-Simulink Converter  PhysicalDomain=network_engine_domain  SubClassName=ps_output  LeftPortType=input  RightPortType=output  PseudoPeriodic=off  Frequencies=[]  VectorFormat=1-D array  Unit=V  AffineConversion=off
      settings: LibrarySourceBlock=SimscapeFPGAHIL_lib/Linearized Switch Models/Switch/vs_out
  + : PMIOPort  Side=Left
  - : PMIOPort  Port=2  Side=Right
  wires:
  Controller/1(ic) -> ic_in/1
  G/1 -> Controller/3(G)
  is_out/1 -> Controller/2(is)
  vs_out/1 -> Controller/1(vs)
  connections:
  is_out/LConn1 -- is/RConn1
  vs_out/LConn1 -- vs/RConn1
  ic_in/RConn1 -- ic/RConn1
  is/LConn1 -- +/RConn1 -- vs/LConn1
  ic/RConn2 -- Gs/RConn1 -- -/RConn1 -- vs/RConn2
  is/RConn2 -- Gs/LConn1 -- ic/LConn1

== system TwoLevelConverterIdealExample_Pejovic/Inverter/Pejovic w//SCA/Switch2 ==
  G : Inport
  Controller : Subsystem  mask{threshold=threshold, Gs=Gs, s=timeScaling, avgFactor=avgFactor}
      mask prompts: Gs "Conductance (1/Ohm)"; s "Time scaling"; avgFactor "Subcycle average factor"
      mask DialogControl DescGroupVar Prompt: Description
      mask DialogControl Details Prompt: Switch Controller
  Gs : fl_lib/Electrical/Electrical Elements/Resistor  R=1/Gs Ohm  i_specify=off  i_priority=None  i=0 A  i_nominal_specify=off  i_nominal_unit=A  i_nominal_value=1  v_specify=off  v_priority=None  v=0 V  v_nominal_specify=off  v_nominal_unit=V  v_nominal_value=1
      settings: LibrarySourceBlock=SimscapeFPGAHIL_lib/Linearized Switch Models/Switch/Gs
  ic : fl_lib/Electrical/Electrical Sources/Controlled Current Source
      settings: LibrarySourceBlock=SimscapeFPGAHIL_lib/Linearized Switch Models/Switch/ic
  ic_in : nesl_utility/Simulink-PS Converter  PhysicalDomain=network_engine_domain  SubClassName=ps_input  LeftPortType=input  RightPortType=output  PseudoPeriodic=off  Frequencies=[]  NoiseDistribution=none  NoiseParameters=[]  Unit=A  AffineConversion=off  FilteringAndDerivatives=provide  SimscapeFilterOrder=1  InputFilterTimeConstant=0.001  UdotUserProvided=0
      settings: LibrarySourceBlock=SimscapeFPGAHIL_lib/Linearized Switch Models/Switch/ic_in
  is : fl_lib/Electrical/Electrical Sensors/Current Sensor
      settings: LibrarySourceBlock=SimscapeFPGAHIL_lib/Linearized Switch Models/Switch/is
  is_out : nesl_utility/PS-Simulink Converter  PhysicalDomain=network_engine_domain  SubClassName=ps_output  LeftPortType=input  RightPortType=output  PseudoPeriodic=off  Frequencies=[]  VectorFormat=1-D array  Unit=A  AffineConversion=off
      settings: LibrarySourceBlock=SimscapeFPGAHIL_lib/Linearized Switch Models/Switch/is_out
  vs : fl_lib/Electrical/Electrical Sensors/Voltage Sensor
      settings: LibrarySourceBlock=SimscapeFPGAHIL_lib/Linearized Switch Models/Switch/vs
  vs_out : nesl_utility/PS-Simulink Converter  PhysicalDomain=network_engine_domain  SubClassName=ps_output  LeftPortType=input  RightPortType=output  PseudoPeriodic=off  Frequencies=[]  VectorFormat=1-D array  Unit=V  AffineConversion=off
      settings: LibrarySourceBlock=SimscapeFPGAHIL_lib/Linearized Switch Models/Switch/vs_out
  + : PMIOPort  Side=Left
  - : PMIOPort  Port=2  Side=Right
  wires:
  vs_out/1 -> Controller/1(vs)
  is_out/1 -> Controller/2(is)
  G/1 -> Controller/3(G)
  Controller/1(ic) -> ic_in/1
  connections:
  ic/LConn1 -- Gs/LConn1 -- is/RConn2
  vs/RConn2 -- -/RConn1 -- Gs/RConn1 -- ic/RConn2
  vs/LConn1 -- +/RConn1 -- is/LConn1
  ic_in/RConn1 -- ic/RConn1
  vs_out/LConn1 -- vs/RConn1
  is_out/LConn1 -- is/RConn1

== system TwoLevelConverterIdealExample_Pejovic/Inverter/Pejovic w//SCA/Switch3 ==
  G : Inport
  Controller : Subsystem  mask{threshold=threshold, Gs=Gs, s=timeScaling, avgFactor=avgFactor}
      mask prompts: Gs "Conductance (1/Ohm)"; s "Time scaling"; avgFactor "Subcycle average factor"
      mask DialogControl DescGroupVar Prompt: Description
      mask DialogControl Details Prompt: Switch Controller
  Gs : fl_lib/Electrical/Electrical Elements/Resistor  R=1/Gs Ohm  i_specify=off  i_priority=None  i=0 A  i_nominal_specify=off  i_nominal_unit=A  i_nominal_value=1  v_specify=off  v_priority=None  v=0 V  v_nominal_specify=off  v_nominal_unit=V  v_nominal_value=1
      settings: LibrarySourceBlock=SimscapeFPGAHIL_lib/Linearized Switch Models/Switch/Gs
  ic : fl_lib/Electrical/Electrical Sources/Controlled Current Source
      settings: LibrarySourceBlock=SimscapeFPGAHIL_lib/Linearized Switch Models/Switch/ic
  ic_in : nesl_utility/Simulink-PS Converter  PhysicalDomain=network_engine_domain  SubClassName=ps_input  LeftPortType=input  RightPortType=output  PseudoPeriodic=off  Frequencies=[]  NoiseDistribution=none  NoiseParameters=[]  Unit=A  AffineConversion=off  FilteringAndDerivatives=provide  SimscapeFilterOrder=1  InputFilterTimeConstant=0.001  UdotUserProvided=0
      settings: LibrarySourceBlock=SimscapeFPGAHIL_lib/Linearized Switch Models/Switch/ic_in
  is : fl_lib/Electrical/Electrical Sensors/Current Sensor
      settings: LibrarySourceBlock=SimscapeFPGAHIL_lib/Linearized Switch Models/Switch/is
  is_out : nesl_utility/PS-Simulink Converter  PhysicalDomain=network_engine_domain  SubClassName=ps_output  LeftPortType=input  RightPortType=output  PseudoPeriodic=off  Frequencies=[]  VectorFormat=1-D array  Unit=A  AffineConversion=off
      settings: LibrarySourceBlock=SimscapeFPGAHIL_lib/Linearized Switch Models/Switch/is_out
  vs : fl_lib/Electrical/Electrical Sensors/Voltage Sensor
      settings: LibrarySourceBlock=SimscapeFPGAHIL_lib/Linearized Switch Models/Switch/vs
  vs_out : nesl_utility/PS-Simulink Converter  PhysicalDomain=network_engine_domain  SubClassName=ps_output  LeftPortType=input  RightPortType=output  PseudoPeriodic=off  Frequencies=[]  VectorFormat=1-D array  Unit=V  AffineConversion=off
      settings: LibrarySourceBlock=SimscapeFPGAHIL_lib/Linearized Switch Models/Switch/vs_out
  + : PMIOPort  Side=Left
  - : PMIOPort  Port=2  Side=Right
  wires:
  Controller/1(ic) -> ic_in/1
  G/1 -> Controller/3(G)
  is_out/1 -> Controller/2(is)
  vs_out/1 -> Controller/1(vs)
  connections:
  is_out/LConn1 -- is/RConn1
  vs_out/LConn1 -- vs/RConn1
  ic_in/RConn1 -- ic/RConn1
  is/LConn1 -- +/RConn1 -- vs/LConn1
  ic/RConn2 -- Gs/RConn1 -- -/RConn1 -- vs/RConn2
  is/RConn2 -- Gs/LConn1 -- ic/LConn1

== system TwoLevelConverterIdealExample_Pejovic/Inverter/Pejovic w//SCA/Switch4 ==
  G : Inport
  Controller : Subsystem  mask{threshold=threshold, Gs=Gs, s=timeScaling, avgFactor=avgFactor}
      mask prompts: Gs "Conductance (1/Ohm)"; s "Time scaling"; avgFactor "Subcycle average factor"
      mask DialogControl DescGroupVar Prompt: Description
      mask DialogControl Details Prompt: Switch Controller
  Gs : fl_lib/Electrical/Electrical Elements/Resistor  R=1/Gs Ohm  i_specify=off  i_priority=None  i=0 A  i_nominal_specify=off  i_nominal_unit=A  i_nominal_value=1  v_specify=off  v_priority=None  v=0 V  v_nominal_specify=off  v_nominal_unit=V  v_nominal_value=1
      settings: LibrarySourceBlock=SimscapeFPGAHIL_lib/Linearized Switch Models/Switch/Gs
  ic : fl_lib/Electrical/Electrical Sources/Controlled Current Source
      settings: LibrarySourceBlock=SimscapeFPGAHIL_lib/Linearized Switch Models/Switch/ic
  ic_in : nesl_utility/Simulink-PS Converter  PhysicalDomain=network_engine_domain  SubClassName=ps_input  LeftPortType=input  RightPortType=output  PseudoPeriodic=off  Frequencies=[]  NoiseDistribution=none  NoiseParameters=[]  Unit=A  AffineConversion=off  FilteringAndDerivatives=provide  SimscapeFilterOrder=1  InputFilterTimeConstant=0.001  UdotUserProvided=0
      settings: LibrarySourceBlock=SimscapeFPGAHIL_lib/Linearized Switch Models/Switch/ic_in
  is : fl_lib/Electrical/Electrical Sensors/Current Sensor
      settings: LibrarySourceBlock=SimscapeFPGAHIL_lib/Linearized Switch Models/Switch/is
  is_out : nesl_utility/PS-Simulink Converter  PhysicalDomain=network_engine_domain  SubClassName=ps_output  LeftPortType=input  RightPortType=output  PseudoPeriodic=off  Frequencies=[]  VectorFormat=1-D array  Unit=A  AffineConversion=off
      settings: LibrarySourceBlock=SimscapeFPGAHIL_lib/Linearized Switch Models/Switch/is_out
  vs : fl_lib/Electrical/Electrical Sensors/Voltage Sensor
      settings: LibrarySourceBlock=SimscapeFPGAHIL_lib/Linearized Switch Models/Switch/vs
  vs_out : nesl_utility/PS-Simulink Converter  PhysicalDomain=network_engine_domain  SubClassName=ps_output  LeftPortType=input  RightPortType=output  PseudoPeriodic=off  Frequencies=[]  VectorFormat=1-D array  Unit=V  AffineConversion=off
      settings: LibrarySourceBlock=SimscapeFPGAHIL_lib/Linearized Switch Models/Switch/vs_out
  + : PMIOPort  Side=Left
  - : PMIOPort  Port=2  Side=Right
  wires:
  vs_out/1 -> Controller/1(vs)
  is_out/1 -> Controller/2(is)
  G/1 -> Controller/3(G)
  Controller/1(ic) -> ic_in/1
  connections:
  ic/LConn1 -- Gs/LConn1 -- is/RConn2
  vs/RConn2 -- -/RConn1 -- Gs/RConn1 -- ic/RConn2
  vs/LConn1 -- +/RConn1 -- is/LConn1
  ic_in/RConn1 -- ic/RConn1
  vs_out/LConn1 -- vs/RConn1
  is_out/LConn1 -- is/RConn1

== system TwoLevelConverterIdealExample_Pejovic/Inverter/Pejovic w//SCA/Switch5 ==
  G : Inport
  Controller : Subsystem  mask{threshold=threshold, Gs=Gs, s=timeScaling, avgFactor=avgFactor}
      mask prompts: Gs "Conductance (1/Ohm)"; s "Time scaling"; avgFactor "Subcycle average factor"
      mask DialogControl DescGroupVar Prompt: Description
      mask DialogControl Details Prompt: Switch Controller
  Gs : fl_lib/Electrical/Electrical Elements/Resistor  R=1/Gs Ohm  i_specify=off  i_priority=None  i=0 A  i_nominal_specify=off  i_nominal_unit=A  i_nominal_value=1  v_specify=off  v_priority=None  v=0 V  v_nominal_specify=off  v_nominal_unit=V  v_nominal_value=1
      settings: LibrarySourceBlock=SimscapeFPGAHIL_lib/Linearized Switch Models/Switch/Gs
  ic : fl_lib/Electrical/Electrical Sources/Controlled Current Source
      settings: LibrarySourceBlock=SimscapeFPGAHIL_lib/Linearized Switch Models/Switch/ic
  ic_in : nesl_utility/Simulink-PS Converter  PhysicalDomain=network_engine_domain  SubClassName=ps_input  LeftPortType=input  RightPortType=output  PseudoPeriodic=off  Frequencies=[]  NoiseDistribution=none  NoiseParameters=[]  Unit=A  AffineConversion=off  FilteringAndDerivatives=provide  SimscapeFilterOrder=1  InputFilterTimeConstant=0.001  UdotUserProvided=0
      settings: LibrarySourceBlock=SimscapeFPGAHIL_lib/Linearized Switch Models/Switch/ic_in
  is : fl_lib/Electrical/Electrical Sensors/Current Sensor
      settings: LibrarySourceBlock=SimscapeFPGAHIL_lib/Linearized Switch Models/Switch/is
  is_out : nesl_utility/PS-Simulink Converter  PhysicalDomain=network_engine_domain  SubClassName=ps_output  LeftPortType=input  RightPortType=output  PseudoPeriodic=off  Frequencies=[]  VectorFormat=1-D array  Unit=A  AffineConversion=off
      settings: LibrarySourceBlock=SimscapeFPGAHIL_lib/Linearized Switch Models/Switch/is_out
  vs : fl_lib/Electrical/Electrical Sensors/Voltage Sensor
      settings: LibrarySourceBlock=SimscapeFPGAHIL_lib/Linearized Switch Models/Switch/vs
  vs_out : nesl_utility/PS-Simulink Converter  PhysicalDomain=network_engine_domain  SubClassName=ps_output  LeftPortType=input  RightPortType=output  PseudoPeriodic=off  Frequencies=[]  VectorFormat=1-D array  Unit=V  AffineConversion=off
      settings: LibrarySourceBlock=SimscapeFPGAHIL_lib/Linearized Switch Models/Switch/vs_out
  + : PMIOPort  Side=Left
  - : PMIOPort  Port=2  Side=Right
  wires:
  Controller/1(ic) -> ic_in/1
  G/1 -> Controller/3(G)
  is_out/1 -> Controller/2(is)
  vs_out/1 -> Controller/1(vs)
  connections:
  is_out/LConn1 -- is/RConn1
  vs_out/LConn1 -- vs/RConn1
  ic_in/RConn1 -- ic/RConn1
  is/LConn1 -- +/RConn1 -- vs/LConn1
  ic/RConn2 -- Gs/RConn1 -- -/RConn1 -- vs/RConn2
  is/RConn2 -- Gs/LConn1 -- ic/LConn1
